simulink library "hddc_lib"  (Simulink 8.7)
settings: Solver=ode45  StartTime=0.0  StopTime=10.0  RelTol=1e-3
undefined symbols (not defined in the file): display, value
libraries: DSPBAPrim x6, DSPBABase x4, DSPBAFilters x4
settings Model: Creator=bigcat  LastModifiedBy=5g

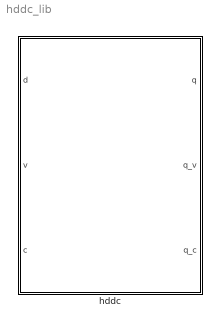
== system hddc_lib ==
  hddc : Subsystem  mask{Clock_Margin=0, HB7_filter_SampleRate=0, HB7_filter_Decimation=0, HB7_filter_ChanCount=0, HB7_filter_coeffs=0, HB7_filter_base_addr=0, HB6_filter_SampleRate=0, HB6_filter_Decimation=0, HB6_filter_ChanCount=0, HB6_filter_coeffs=0, HB6_filter_base_addr=0, output_word_length=0, output_fraction_length=0}
      mask Display:
      | disp('HDDC');
      | port_label('input',1,'d');
      | port_label('input',2,'v');
      | port_label('input',3,'c');
      | port_label('output',1,'q');
      | port_label('output',2,'q_v');
      | port_label('output',3,'q_c');

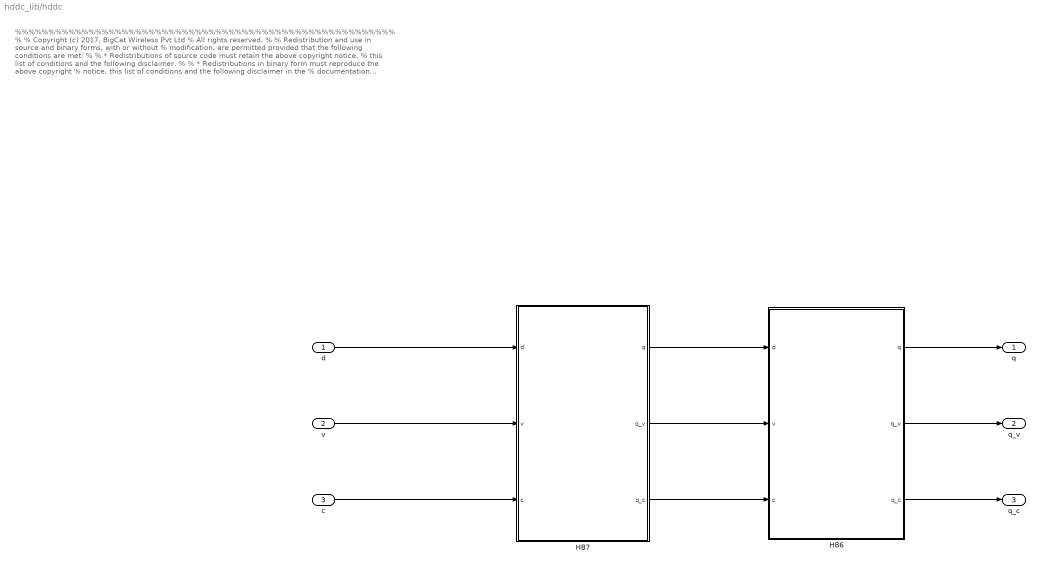
== system hddc_lib/hddc ==
  note: %%%%%%%%%%%%%%%%%%%%%%%%%%%%%%%%%%%%%%%%%%%%%%%%%%%%%%%%%
      |  %
      |  % Copyright (c) 2017, BigCat Wireless Pvt Ltd
      |  % All rights reserved.
      |  %
      |  % Redistribution and use in source and binary forms, with or without
      |  % modification, are permitted provided that the following conditions are met:
      |  %
      |  %     * Redistributions of source code must retain the above copyright notice,
      |  %       this list of conditions and the following disclaimer.
      |  %
      |  %     * Redistributions in binary form must reproduce the above copyright
      |  %       notice, this list of conditions and the following disclaimer in the
      |  %       documentation and/or other materials provided with the distribution.
      |  %
      |  %     * Neither the name of the copyright holder nor the names of its contributors
      |  %       may be used to endorse or promote products derived from this software
      |  %       without specific prior written permission.
      |  %
      |  %
      |  %
      |  % THIS SOFTWARE IS PROVIDED BY THE COPYRIGHT HOLDERS AND CONTRIBUTORS "AS IS"
      |  % AND ANY EXPRESS OR IMPLIED WARRANTIES, INCLUDING, BUT NOT LIMITED TO, THE
      |  % IMPLIED WARRANTIES OF MERCHANTABILITY AND FITNESS FOR A PARTICULAR PURPOSE ARE
      |  % DISCLAIMED. IN NO EVENT SHALL THE COPYRIGHT HOLDER OR CONTRIBUTORS BE LIABLE
      |  % FOR ANY DIRECT, INDIRECT, INCIDENTAL, SPECIAL, EXEMPLARY, OR CONSEQUENTIAL
      |  % DAMAGES (INCLUDING, BUT NOT LIMITED TO, PROCUREMENT OF SUBSTITUTE GOODS OR
      |  % SERVICES; LOSS OF USE, DATA, OR PROFITS; OR BUSINESS INTERRUPTION) HOWEVER
      |  % CAUSED AND ON ANY THEORY OF LIABILITY, WHETHER IN CONTRACT, STRICT LIABILITY,
      |  % OR TORT (INCLUDING NEGLIGENCE OR OTHERWISE) ARISING IN ANY WAY OUT OF THE USE
      |  % OF THIS SOFTWARE, EVEN IF ADVISED OF THE POSSIBILITY OF SUCH DAMAGE.
      |  %
      |   %%%%%%%%%%%%%%%%%%%%%%%%%%%%%%%%%%%%%%%%%%%%%%%%%%%%%%%%%%
  d : Inport
  v : Inport  Port=2
  c : Inport  Port=3
  HB6 : Subsystem
  HB7 : Subsystem
  q : Outport
  q_v : Outport  Port=2
  q_c : Outport  Port=3
  wires:
  HB6/3(q_c) -> q_c/1
  v/1 -> HB7/2(v)
  c/1 -> HB7/3(c)
  HB6/1(q) -> q/1
  HB6/2(q_v) -> q_v/1
  HB7/1(q) -> HB6/1(d)
  HB7/2(q_v) -> HB6/2(v)
  d/1 -> HB7/1(d)
  HB7/3(q_c) -> HB6/3(c)

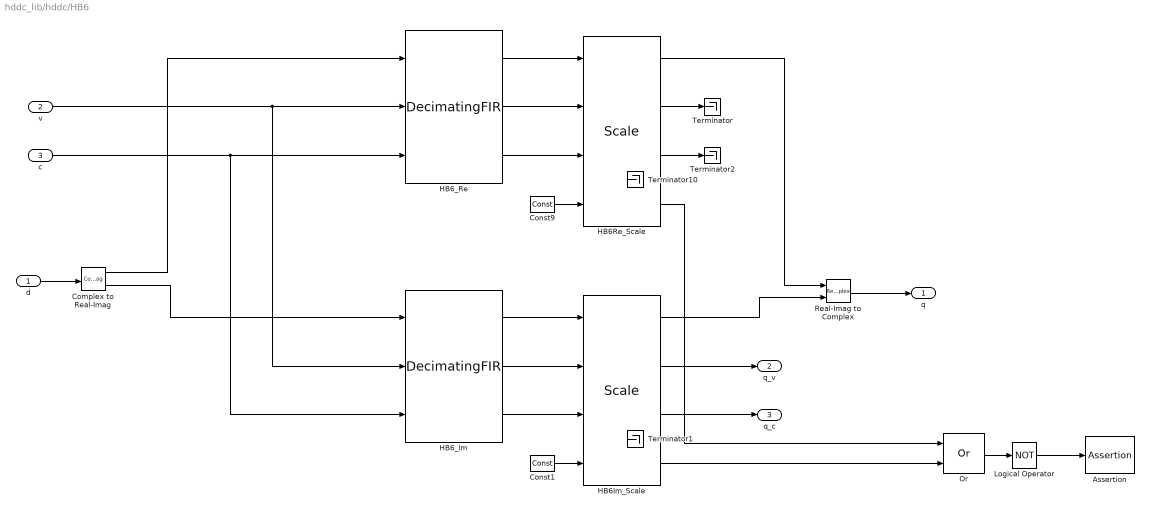
== system hddc_lib/hddc/HB6 ==
  d : Inport
  v : Inport  Port=2
  c : Inport  Port=3
  Assertion : Assertion  Enabled=off  AssertionFailFcn=display('Simulation stopped, because an over/underflow was detected in HDDC/HB7')
  Complex to Real-Imag : ComplexToRealImag
  Const1 : DSPBAPrim/Const  primtype=const  nInputs=0  nOutputs=1  omode=Inherit via internal rule  otype=sfix(16)  scale=2^-15  rndmethod=Unbiased  factor=1  satmethod=Symmetric  shift_vec=[0 1 2 -1]  value=0  inPortNames=['+'; '+';]  outPortNames=[' ']  dspbaimage=dspba_prim.jpg  text=fprintf('%s', num2str(value));  style=Optimised  visibilities=8 + 1024  floatPrecision=float32_m23  version=20120820
  Const9 : DSPBAPrim/Const  primtype=const  nInputs=0  nOutputs=1  omode=Inherit via internal rule  otype=sfix(16)  scale=2^-15  rndmethod=Unbiased  factor=1  satmethod=Symmetric  shift_vec=[0 1 2 -1]  value=0  inPortNames=['+'; '+';]  outPortNames=[' ']  dspbaimage=dspba_prim.jpg  text=fprintf('%s', num2str(value));  style=Optimised  visibilities=8 + 1024  floatPrecision=float32_m23  version=20120820
  HB6Im_Scale : DSPBABase/Scale  otype=sfix(output_word_length)  scale=2^-output_fraction_length  rndmethod=Truncate  factor=1  satmethod=Symmetric  shift_vec=0  latency=4  wideSimulation=off  version=20130807
  HB6Re_Scale : DSPBABase/Scale  otype=sfix(output_word_length)  scale=2^-output_fraction_length  rndmethod=Truncate  factor=1  satmethod=Symmetric  shift_vec=0  latency=4  wideSimulation=off  version=20130807
  HB6_Im : DSPBAFilters/DecimatingFIR  nInputRate=HB6_filter_SampleRate  decim=HB6_filter_Decimation  nchan=HB6_filter_ChanCount  symmetry=Symmetrical  coef=HB6_filter_coeffs  addr=HB6_filter_base_addr  rwmode=Constant  nband=Half Band  exposebus=off  latency=24  version=20090407  recon=off  MM=[0,1,2,3,4,5,6,7,8,9,10,11,12,13,14,15]
  HB6_Re : DSPBAFilters/DecimatingFIR  nInputRate=HB6_filter_SampleRate  decim=HB6_filter_Decimation  nchan=HB6_filter_ChanCount  symmetry=Symmetrical  coef=HB6_filter_coeffs  addr=HB6_filter_base_addr  rwmode=Constant  nband=Half Band  exposebus=off  latency=24  version=20090407  recon=off  MM=[0,1,2,3,4,5,6,7,8,9,10,11,12,13,14,15]
  Logical Operator : Logic  Operator=NOT  Inputs=1  AllPortsSameDT=off  OutDataTypeStr=boolean
  Or : DSPBAPrim/Or  primtype=or  nInputs=2  nOutputs=1  omode=Inherit via internal rule  otype=sfix(16)  scale=2^-15  rndmethod=Unbiased  factor=1  satmethod=Symmetric  shift_vec=[0 1 2 -1]  value=0  inPortNames=[' '; ' '; ' '; ' '; ' '; ' '; ' '; ' '; ' '; ' '; ' '; ' '; ' '; ' '; ' '; ' '; ]  outPortNames=[' ']  dspbaimage=dspba_prim.jpg  text=fprintf('|');  style=Optimised  visibilities=8+2  version=20090407
  Real-Imag to Complex : RealImagToComplex
  Terminator{,1..2,10} (4 alike) : Terminator
  q : Outport
  q_v : Outport  Port=2
  q_c : Outport  Port=3
  wires:
  HB6_Re/3 -> HB6Re_Scale/3
  HB6_Re/1 -> HB6Re_Scale/1
  HB6_Re/2 -> HB6Re_Scale/2
  Const9/1 -> HB6Re_Scale/4
  HB6Re_Scale/4 -> Or/1
  HB6_Im/3 -> HB6Im_Scale/3
  HB6_Im/1 -> HB6Im_Scale/1
  HB6_Im/2 -> HB6Im_Scale/2
  Const1/1 -> HB6Im_Scale/4
  HB6Im_Scale/4 -> Or/2
  v/1 -> HB6_Im/2, HB6_Re/2
  c/1 -> HB6_Im/3, HB6_Re/3
  Complex to Real-Imag/2 -> HB6_Im/1
  HB6Im_Scale/1 -> Real-Imag to Complex/2
  HB6Im_Scale/3 -> q_c/1
  HB6Im_Scale/2 -> q_v/1
  Or/1 -> Logical Operator/1
  Logical Operator/1 -> Assertion/1
  d/1 -> Complex to Real-Imag/1
  Complex to Real-Imag/1 -> HB6_Re/1
  HB6Re_Scale/1 -> Real-Imag to Complex/1
  Real-Imag to Complex/1 -> q/1
  HB6Re_Scale/2 -> Terminator/1
  HB6Re_Scale/3 -> Terminator2/1

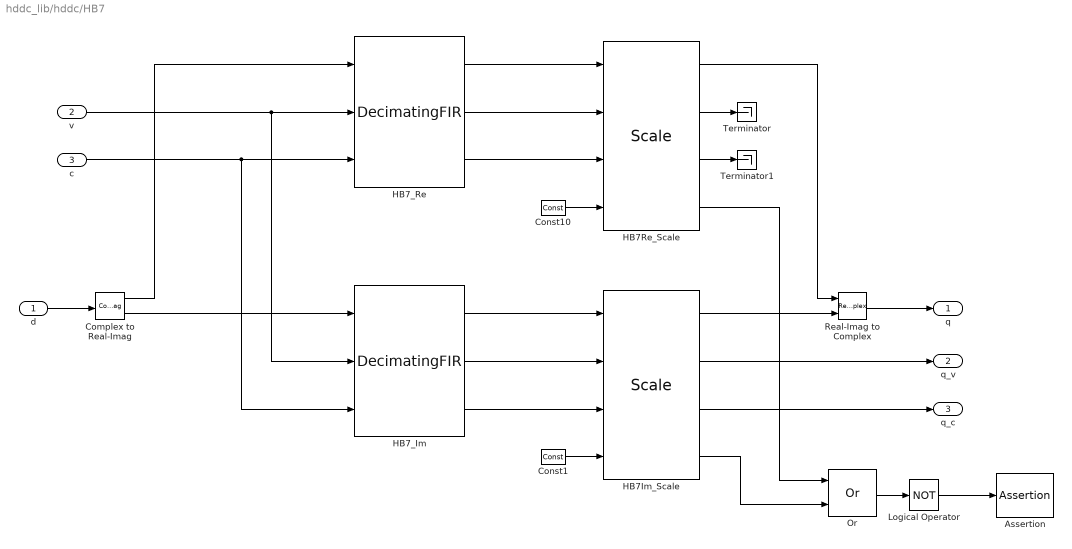
== system hddc_lib/hddc/HB7 ==
  d : Inport
  v : Inport  Port=2
  c : Inport  Port=3
  Assertion : Assertion  Enabled=off  AssertionFailFcn=display('Simulation stopped, because an over/underflow was detected in HDDC/HB7')
  Complex to Real-Imag : ComplexToRealImag
  Const1 : DSPBAPrim/Const  primtype=const  nInputs=0  nOutputs=1  omode=Inherit via internal rule  otype=sfix(16)  scale=2^-15  rndmethod=Unbiased  factor=1  satmethod=Symmetric  shift_vec=[0 1 2 -1]  value=0  inPortNames=['+'; '+';]  outPortNames=[' ']  dspbaimage=dspba_prim.jpg  text=fprintf('%s', num2str(value));  style=Optimised  visibilities=8 + 1024  floatPrecision=float32_m23  version=20120820
  Const10 : DSPBAPrim/Const  primtype=const  nInputs=0  nOutputs=1  omode=Inherit via internal rule  otype=sfix(16)  scale=2^-15  rndmethod=Unbiased  factor=1  satmethod=Symmetric  shift_vec=[0 1 2 -1]  value=0  inPortNames=['+'; '+';]  outPortNames=[' ']  dspbaimage=dspba_prim.jpg  text=fprintf('%s', num2str(value));  style=Optimised  visibilities=8 + 1024  floatPrecision=float32_m23  version=20120820
  HB7Im_Scale : DSPBABase/Scale  otype=sfix(output_word_length)  scale=2^-output_fraction_length  rndmethod=Truncate  factor=1  satmethod=Symmetric  shift_vec=0  latency=4  wideSimulation=off  version=20130807
  HB7Re_Scale : DSPBABase/Scale  otype=sfix(output_word_length)  scale=2^-output_fraction_length  rndmethod=Truncate  factor=1  satmethod=Symmetric  shift_vec=0  latency=4  wideSimulation=off  version=20130807
  HB7_Im : DSPBAFilters/DecimatingFIR  nInputRate=HB7_filter_SampleRate  decim=HB7_filter_Decimation  nchan=HB7_filter_ChanCount  symmetry=Symmetrical  coef=HB7_filter_coeffs  addr=HB7_filter_base_addr  rwmode=Constant  nband=Half Band  exposebus=off  latency=20  version=20090407  recon=off  MM=[0,1,2,3,4,5,6,7,8,9,10,11,12,13,14,15]
  HB7_Re : DSPBAFilters/DecimatingFIR  nInputRate=HB7_filter_SampleRate  decim=HB7_filter_Decimation  nchan=HB7_filter_ChanCount  symmetry=Symmetrical  coef=HB7_filter_coeffs  addr=HB7_filter_base_addr  rwmode=Constant  nband=Half Band  exposebus=off  latency=20  version=20090407  recon=off  MM=[0,1,2,3,4,5,6,7,8,9,10,11,12,13,14,15]
  Logical Operator : Logic  Operator=NOT  Inputs=1  AllPortsSameDT=off  OutDataTypeStr=boolean
  Or : DSPBAPrim/Or  primtype=or  nInputs=2  nOutputs=1  omode=Inherit via internal rule  otype=sfix(16)  scale=2^-15  rndmethod=Unbiased  factor=1  satmethod=Symmetric  shift_vec=[0 1 2 -1]  value=0  inPortNames=[' '; ' '; ' '; ' '; ' '; ' '; ' '; ' '; ' '; ' '; ' '; ' '; ' '; ' '; ' '; ' '; ]  outPortNames=[' ']  dspbaimage=dspba_prim.jpg  text=fprintf('|');  style=Optimised  visibilities=8+2  version=20090407
  Real-Imag to Complex : RealImagToComplex
  Terminator : Terminator
  Terminator1 : Terminator
  q : Outport
  q_v : Outport  Port=2
  q_c : Outport  Port=3
  wires:
  HB7Re_Scale/4 -> Or/1
  HB7_Re/3 -> HB7Re_Scale/3
  HB7_Re/2 -> HB7Re_Scale/2
  Const10/1 -> HB7Re_Scale/4
  HB7_Re/1 -> HB7Re_Scale/1
  HB7Im_Scale/4 -> Or/2
  HB7_Im/3 -> HB7Im_Scale/3
  HB7_Im/2 -> HB7Im_Scale/2
  Const1/1 -> HB7Im_Scale/4
  HB7_Im/1 -> HB7Im_Scale/1
  HB7Im_Scale/1 -> Real-Imag to Complex/2
  v/1 -> HB7_Im/2, HB7_Re/2
  c/1 -> HB7_Im/3, HB7_Re/3
  Complex to Real-Imag/2 -> HB7_Im/1
  d/1 -> Complex to Real-Imag/1
  Complex to Real-Imag/1 -> HB7_Re/1
  HB7Im_Scale/2 -> q_v/1
  HB7Im_Scale/3 -> q_c/1
  Real-Imag to Complex/1 -> q/1
  HB7Re_Scale/1 -> Real-Imag to Complex/1
  HB7Re_Scale/2 -> Terminator/1
  HB7Re_Scale/3 -> Terminator1/1
  Or/1 -> Logical Operator/1
  Logical Operator/1 -> Assertion/1
